simulink model "lin_master_s32k14x"  (Simulink 9.0)
settings: Solver=FixedStepDiscrete  StartTime=0.0  StopTime=10.0  FixedStep=1  RelTol=1e-3  EnableMultiTasking=on
InitFcn:
  | mbd_s32k_consistency_checks(bdroot(gcs));
undefined symbols (not defined in the file): LQFP, send
libraries: mbd_s32k1xx_ec_toolbox x6, simulink x1
Description:
  | Basic example for demonstrating LIN blocks function. The demo requires 2 boards, one running the code from this model, one running the code from the slave model.
  | 
  | Master sends header with ID=1 [PID automatically calculated].
  | This triggers a callback, handled by LIN Callback block.
  | When the ISR is triggered, event (LIN_PID_OK/LIN_PID_ERROR/LIN_CHECKSUM_ERROR/etc) and frameID are passed to the subsystem that is to be called.
  | This way, you can handle all events from all the participants on the LIN bus here.
  | 
  | In this example, after sending the header, the master will send data (6B, having the following format):
  | [0]: inc - a variable that is incremented every second in the main loop
  | [1]: event
  | [2]: frame id
  | [3]: 4 (constant value)
  | [4]: 4 (constant value)
  | [5]: 4 (constant value)
  | 
  | The red LED is toggled on every callback (after each time the master has sent data).
  | 
  | Hardware connections:
  | - external power is needed as VBAT signal is connected to VSUP
  | - wiring:
  | 
  |        |MASTER        -         SLAVE|
  |        |______________________|
  |        |GND             -    GND        |
  |        |LIN[J11.1]      -    LIN[J11.1]  |
  | 
  | Validation:
  | - There is a FreeMASTER project asociated with the slave model - open it and check if the slave receives the data described above.
settings Model: Creator=NXP MBDT Team  LastModifiedBy=nxf35172
settings DataIOCC: ExternalInput=off  InitialState=off  LimitDataPoints=on  SaveOutput=off  SignalLogging=off  SaveTime=off
settings OptimizationCC: DefaultParameterBehavior=Inlined  PassReuseOutputArgsAs=Individual arguments  LifeSpan=auto
settings DebuggingCC: SolverPrmCheckMsg=warning  InheritedTsInSrcMsg=none  SingleTaskRateTransMsg=error  ParameterTunabilityLossMsg=error  UnconnectedInputMsg=error  UnconnectedOutputMsg=error  UnconnectedLineMsg=error  AllowSymbolicDim=off  UnknownTsInhSupMsg=error  StateNameClashWarn=warning
settings HardwareCC: ProdLargestAtomicInteger=Long  ProdLargestAtomicFloat=Double  ProdEndianess=LittleEndian  ProdHWDeviceType=ARM Compatible->ARM Cortex
settings SFSimCC: MATLABDynamicMemAlloc=off
settings RTWCC: SystemTargetFile=mbd_s32k.tlc  MakeCommand=mbd_s32k_make_rtw COPY_MDLREF_INCLUDES=0  TemplateMakefile=mbd_s32k.tmf  Description=Model Based Design Toolbox S32K14x Code Generation Target  GenerateReport=on  IncludeHyperlinkInReport=on  LaunchReport=on  GenerateTraceInfo=on  GenerateTraceReport=on  GenerateTraceReportSl=on  GenerateTraceReportSf=on  GenerateTraceReportEml=on
settings CodeAppCC: ForceParamTrailComments=on  IgnoreCustomStorageClasses=off  OperatorAnnotations=on  SimulinkDataObjDesc=on  SFDataObjDesc=on  InsertBlockDesc=on  StateflowObjectComments=off
settings STFCustomTargetCC: MultiwordLength=256  ModelReferenceCompliant=off  CombineOutputUpdateFcns=on  ERTCustomFileBanners=on  SupportContinuousTime=off  SupportNonInlinedSFcns=off  RemoveResetFunc=on  MATLABClassNameForMDSCustomization=Simulink.SoftwareTarget.ERTCustomization  GRTInterface=off  SystemTargetFile=mbd_s32k.tlc
settings ERTTargetCC: ModelReferenceCompliant=off  ParMdlRefBuildCompliant=off  CompOptLevelCompliant=off  ConcurrentExecutionCompliant=off  ModelStepFunctionPrototypeControlCompliant=off  CPPClassGenCompliant=off  UseToolchainInfoCompliant=off  InlinedParameterPlacement=NonHierarchical  ERTCustomFileTemplate=example_file_process.tlc

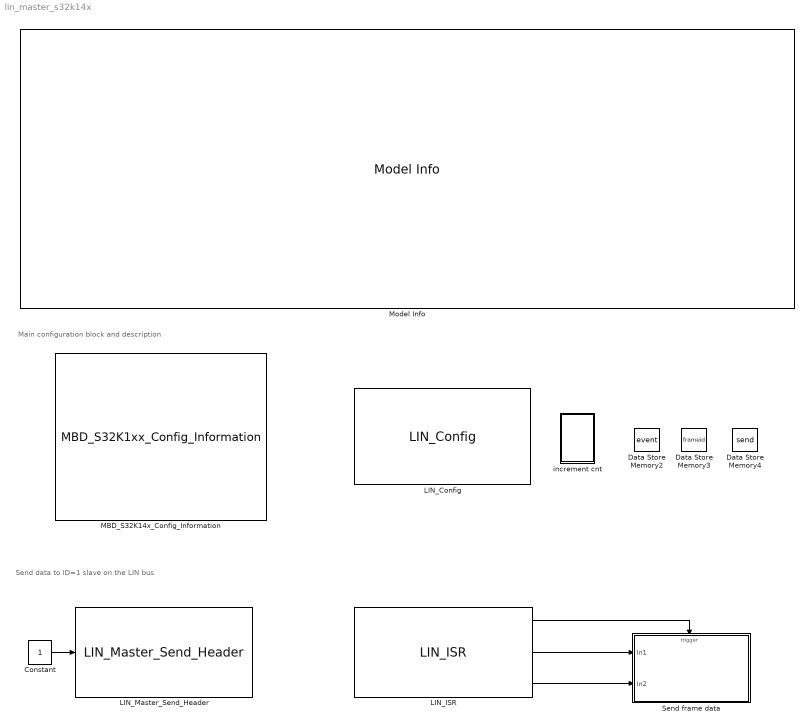
== system lin_master_s32k14x ==
  note: Send data to ID=1 slave on the LIN bus
  note: Main configuration block and description
  Constant : Constant  OutDataTypeStr=uint8
  Data Store Memory2 : DataStoreMemory  DataStoreName=event  ReadBeforeWriteMsg=warning  WriteAfterWriteMsg=warning  WriteAfterReadMsg=warning  ShowAdditionalParam=off  OutDataTypeStr=uint8
  Data Store Memory3 : DataStoreMemory  DataStoreName=frameid  ReadBeforeWriteMsg=warning  WriteAfterWriteMsg=warning  WriteAfterReadMsg=warning  ShowAdditionalParam=off  OutDataTypeStr=uint8
  Data Store Memory4 : DataStoreMemory  DataStoreName=send  ReadBeforeWriteMsg=warning  WriteAfterWriteMsg=warning  WriteAfterReadMsg=warning  InitialValue=[4 4 4 4 4 4]  ShowAdditionalParam=off  OutDataTypeStr=uint8
  LIN_Config : mbd_s32k1xx_ec_toolbox/Communication Blocks/LIN Blocks/LIN_Config  Priority=1  instance=2  baudrate=9600  node_function=MASTER  autobaud_enable=None  rx=PTD6: [LPUART2_RX | Receive]  tx=PTD7: [LPUART2_TX | Transmit]  cts=PTC12: [LPUART2_CTS | Clear To Send (bar)]  rts=PTC13: [LPUART2_RTS | Request To Send]
  LIN_ISR : mbd_s32k1xx_ec_toolbox/Communication Blocks/LIN Blocks/LIN_ISR  instance=2
  LIN_Master_Send_Header : mbd_s32k1xx_ec_toolbox/Communication Blocks/LIN Blocks/LIN_Master_Send_Header  instance=2
  MBD_S32K14x_Config_Information : mbd_s32k1xx_ec_toolbox/MBD_S32K1xx_Config_Information  mbdt_ver=0  disp_str=|  config_params=[]  mcu_target_name=S32K144  mcu_target_package=64-LQFP  mcu_target_sram_size=48KB  mcu_system_clock_freq=80  mcu_xtal_freq=External 8  mcu_steptick_timer=LPIT Channel 0  mcu_steptick_prio=0  ds_import_enable=on  target_compiler=GCC  target_memory=FLASH  gcc_target_compile_opts=-mcpu=cortex-m4 -mthumb -mfloat-abi=hard -mfpu=fpv4-sp-d16 -O1 -g -gstrict-dwarf  gcc_target_assemble_opts=-mcpu=cortex-m4 -mthumb -mfloat-abi=hard -mfpu=fpv4-sp-d16 -g  gcc_target_link_opts=-mcpu=cortex-m4 -mthumb -mfloat-abi=hard -mfpu=fpv4-sp-d16  gcc_target_default_lcf=on  gcc_target_user_lcf=S32K144_48_flash.ld  ghs_target_compile_opts=-cpu=cortexm4f -thumb -DARM_MATH_CM4 -fpu=vfpv4_d16 -fsingle -Ogeneral -Wundef -Wimplicit-int -Wshadow -Wtrigraphs --no_commons --gnu_asm -gnu99 -gdwarf-2 -G  ghs_target_assemble_opts=-cpu=cortexm4f -fpu=vfpv4_d16  ghs_target_link_opts=-cpu=cortexm4f -thumb -fpu=vfpv4_d16  ghs_target_default_lcf=on  ghs_target_user_lcf=S32K144_48_flash.ld  iar_target_compile_opts=--cpu=Cortex-M4F --thumb --fpu=VFPv4_sp -Ol -e --debug --dlib_config normal  iar_target_assemble_opts=--cpu Cortex-M4F --thumb --fpu VFPv4_sp  iar_target_link_opts=--no_exceptions --vfe --inline  iar_target_default_lcf=on  iar_target_user_lcf=S32K144_48_flash.icf  pil_download_enable=off  rbl_download_enable=on  rbl_start_delay=5000000  rbl_download_interface=OpenSDA  rbl_restart_request=off  rbl_com_port=Custom  rbl_com_port_custom=COM1  pil_download_rate=57600  pil_opensda_drive=Custom  pil_opensda_drive_custom=D  pil_uart_instance=0  pil_uart_rx=PTA2: [LPUART0_RX | Receive]  pil_uart_tx=PTA3: [LPUART0_TX | Transmit]  FTM_PWM_PcrCheckEnDis=on  FTM_Input_Edge_Inputs_PcrCheckEnDis=on  FTM_Dual_Edge_Inputs_PcrCheckEnDis=on  FTM_Quadrature_Inputs_PcrCheckEnDis=on  FTM_Hall_Sensor_Inputs_PcrCheckEnDis=on  LPTMR_PcrCheckEnDis=on  PIT_PcrCheckEnDis=on  RTC_PcrCheckEnDis=on  FlexCAN_PcrCheckEnDis=on  LIN_PcrCheckEnDis=on  FlexIO_PcrCheckEnDis=on  LPI2C_PcrCheckEnDis=on  LPSPI_PcrCheckEnDis=on  LPUART_PcrCheckEnDis=on  CMP_PcrCheckEnDis=on  GPIO_OutputPcrCheckEnDis=on  GPIO_InputPcrCheckEnDis=on  SBC_PcrCheckEnDis=on  AMMCLIB_PcrCheckEnDis=on  FM_PcrCheckEnDis=on  Profile_PcrCheckEnDis=on  ConfigParams_PcrCheckEnDis=on  ModelRef_PcrCheckEnDis=on  PDB0_PcrCheckEnDis=on  CSEc_PcrCheckEnDis=off  eDMA_PcrCheckEnDis=on  ADC_PcrCheckEnDis=on  WDOG_PcrCheckEnDis=on
      | Target : S32K144-48KB_SRAM
      | Package : 100-pin
      | System clock : 80 MHz
      | XTAL clock : External 8 MHz
      | Compiler : IAR
      | Target Type : FLASH
      | Download Code after build : off
      | Step Tick Interrupt Priority : 15
  Model Info : simulink/Model-Wide Utilities/Model Info  Frame=on  DisplayStringWithTags=|  HorizontalTextAlignment=Center  LeftAlignmentValue=0.5
      | %<ModelName>
      | %<Description>
  Send frame data : Subsystem  TreatAsAtomicUnit=on
      settings: RTWSystemCode=Nonreusable function
  increment cnt : Subsystem
  wires:
  LIN_ISR/1 -> Send frame data/Trigger
  Constant/1 -> LIN_Master_Send_Header/1
  LIN_ISR/2 -> Send frame data/1(In1)
  LIN_ISR/3 -> Send frame data/2(In2)

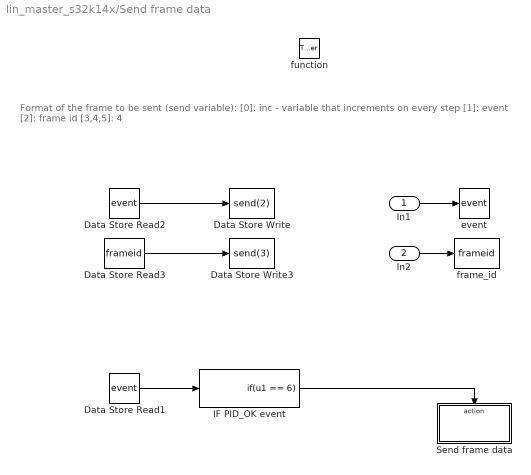
== system lin_master_s32k14x/Send frame data ==
  note: Format of the frame to be sent (send variable):
      | [0]: inc - variable that increments on every step
      | [1]: event
      | [2]: frame id
      | [3,4,5]: 4
  In1 : Inport
  In2 : Inport  Port=2
  function : TriggerPort  TriggerType=function-call  VariantControl=Variant
  Data Store Read1 : DataStoreRead  DataStoreName=event
  Data Store Read2 : DataStoreRead  Priority=2  DataStoreName=event
  Data Store Read3 : DataStoreRead  DataStoreName=frameid
  Data Store Write : DataStoreWrite  Priority=1  DataStoreName=send  DataStoreElements=send(2)
  Data Store Write3 : DataStoreWrite  Priority=1  DataStoreName=send  DataStoreElements=send(3)
  IF PID_OK event : If  IfExpression=u1 == 6  ShowElse=off
  Send frame data : Subsystem  TreatAsAtomicUnit=on
  event : DataStoreWrite  Priority=1  DataStoreName=event
  frame_id : DataStoreWrite  DataStoreName=frameid
  wires:
  In2/1 -> frame_id/1
  In1/1 -> event/1
  Data Store Read2/1 -> Data Store Write/1
  Data Store Read3/1 -> Data Store Write3/1
  IF PID_OK event/1 -> Send frame data/Action
  Data Store Read1/1 -> IF PID_OK event/1

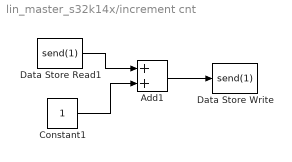
== system lin_master_s32k14x/increment cnt ==
  Add1 : Sum
  Constant1 : Constant  OutDataTypeStr=uint8
  Data Store Read1 : DataStoreRead  DataStoreName=send  DataStoreElements=send(1)
  Data Store Write : DataStoreWrite  DataStoreName=send  DataStoreElements=send(1)
  wires:
  Data Store Read1/1 -> Add1/1
  Constant1/1 -> Add1/2
  Add1/1 -> Data Store Write/1

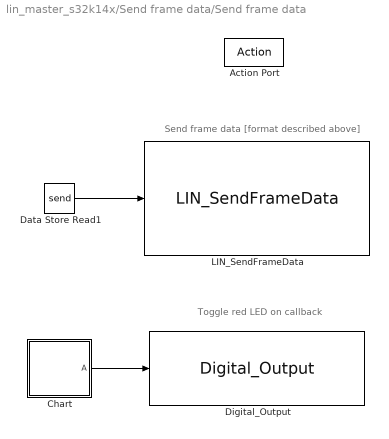
== system lin_master_s32k14x/Send frame data/Send frame data ==
  note: Toggle red LED on callback
  note: Send frame data [format described above]
  Action Port : ActionPort
  Chart : Stateflow chart  TreatAsAtomicUnit=on
  Data Store Read1 : DataStoreRead  Priority=2  DataStoreName=send
  Digital_Output : mbd_s32k1xx_ec_toolbox/GPIO Blocks/Digital_Output  Priority=28  gpio_pin=PTD15: [PTD15 | Port D I/O]  init_val=Low  drive_strength=Low
  LIN_SendFrameData : mbd_s32k1xx_ec_toolbox/Communication Blocks/LIN Blocks/LIN_SendFrameData  Priority=23  instance=2
  wires:
  Chart/1(" A") -> Digital_Output/1
  Data Store Read1/1 -> LIN_SendFrameData/1

== stateflow chart Send frame data/Send frame data/Chart ==
  state A
  state A1
  (default) -> A
  A -> A1
  A1 -> A
  data: A output boolean [0..1]
